simulink model "Demo_MinSegMega_V4"  (R2015a)
settings: Solver=FixedStepDiscrete  SolverMode=SingleTasking  StartTime=0.0  StopTime=inf  FixedStep=.05  RelTol=1e-3
PostLoadFcn:
  | try,
  | codertarget.arduinobase.registry.setBaudRate(gcs,115200)
  | disp('baud rate set to 115200 for external mode hardware serial')
  | baudrate='set_to_115200'
  | catch
  | disp('baud rate setting not needed in this version')
  | end
libraries: arduinolib x8, RASPlib x7, MinSegLibrary_MinSegMega x4
settings Model: SimulationMode=external  ExtModeTrigDuration=2  Creator=Alec  LastModifiedBy=hurstj
settings OptimizationCC: ExpressionDepthLimit=2147483647  OptimizeModelRefInitCode=on  LifeSpan=1
settings DebuggingCC: UnderspecifiedInitializationDetection=Classic  MergeDetectMultiDrivingBlocksExec=none  StateNameClashWarn=warning
settings HardwareCC: ProdBitPerInt=16  ProdBitPerPointer=8  ProdIntDivRoundTo=Zero  ProdEndianess=LittleEndian  ProdWordSize=8  ProdHWDeviceType=Atmel->AVR
settings RTWCC: SystemTargetFile=realtime.tlc  GenerateMakefile=off  TemplateMakefile=realtime.tmf  Description=Real-Time Toolbox  RTWVerbose=off
settings CodeAppCC: CustomSymbolStrType=$N$R$M  InternalIdentifier=Classic
settings ERTTargetCC: CombineOutputUpdateFcns=off  ExtMode=on  ExtModeTransport=3  ExtModeMexArgs=0 45 115200 30  ERTSrcFileBannerTemplate=realtime_code_template.cgt  ERTHdrFileBannerTemplate=realtime_code_template.cgt  ERTDataSrcFileTemplate=realtime_code_template.cgt  ERTDataHdrFileTemplate=realtime_code_template.cgt  ERTCustomFileTemplate=realtime_file_process.tlc

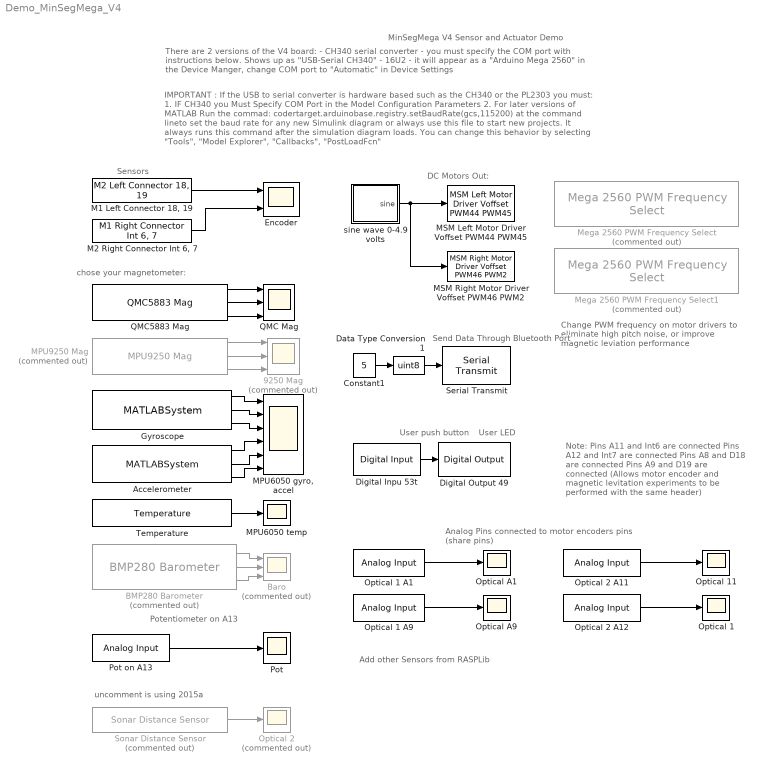
== system Demo_MinSegMega_V4 ==
  note: There are 2 versions of the V4 board:
      | - CH340 serial converter - you must specify the COM port with instructions  below. Shows up as "USB-Serial CH340"
      | - 16U2  - it will appear as a "Arduino Mega 2560" in the Device Manger, change  COM port to  "Automatic" in Device Settings
  note: Change PWM frequency on motor drivers
      | to eliminate high pitch noise, or improve
      | magnetic leviation performance
  note: Add other Sensors from RASPLib
  note: uncomment is using 2015a
  note: MinSegMega V4 Sensor and Actuator Demo
  note: DC Motors Out:
  note: Sensors
  note: Send Data Through Bluetooth Port
  note: User push button
  note: Analog Pins connected to
      | motor encoders pins (share pins)
  note: User LED
  note: Potentiometer on A13
  note: Note: Pins  A11 and Int6 are connected
      |          Pins  A12 and Int7 are connected
      | 	  Pins  A8 and D18 are connected
      |          Pins  A9 and D19 are connected
      | (Allows  motor encoder and magnetic
      | levitation experiments to be performed
      | with the same header)
  note: IMPORTANT : If the USB to serial converter is hardware based such as the CH340 or the PL2303 you must:
      | 1. IF CH340 you Must Specify COM Port in the Model Configuration Parameters
      | 2. For later versions of MATLAB Run the commad: codertarget.arduinobase.registry.setBaudRate(gcs,115200)
      | at the command lineto set the baud rate for any new Simulink diagram or always use this file to start new projects.
      | It always runs this command after the simulation diagram loads.
      | You can change this behavior by selecting "Tools", "Model Explorer", "Callbacks", "PostLoadFcn"
  note: chose your magnetometer:
  9250 Mag : Scope  Commented=on  NumInputPorts=3
      settings: TimeRange=30  YMin=-200~-200~-200  YMax=200~200~200  SaveName=ScopeData7
  Accelerometer : MATLABSystem  System=soMPU6050Accel  SimulateUsing=Code generation
      mask Type: soMPU6050Accel
      mask Display:
      | disp('soMPU6050Accel');
      | port_label('output',1,'xaccel');
      | port_label('output',2,'yaccel');
      | port_label('output',3,'zaccel');
  BMP280 Barometer : RASPlib/BMP280 Barometer  Commented=on  SimulateUsing=Code generation
  Baro : Scope  Commented=on  NumInputPorts=3
      settings: TimeRange=10  YMin=100663~53.25~28.42  YMax=100685~55.25~28.55  SaveName=ScopeData2
  Constant1 : Constant  Value=5  SampleTime=-1
  Data Type Conversion1 : DataTypeConversion  OutDataTypeStr=uint8
  Digital Inpu 53t : arduinolib/Digital Input  pinNumber=53  sampleTime=-1  blockPlatform=arduino
  Digital Output 49 : arduinolib/Digital Output  pinNumber=49  blockPlatform=arduino
  Encoder : Scope  NumInputPorts=2
      settings: TimeRange=30  YMin=-1000~-1000  YMax=1000~1000  ScrollMode=on
  Gyroscope : MATLABSystem  System=soMPU6050Gyro  DLPFmode=0
      mask Type: soMPU6050Gyro
      mask Display:
      | disp('soMPU6050Gyro');
      | port_label('output',1,'xvel');
      | port_label('output',2,'yvel');
      | port_label('output',3,'zvel');
  "M1 Left Connector 18, 19" : MinSegLibrary_MinSegMega/M2 Left Connector 18, 19  Encoder=1  PinA=19  PinB=18
  "M2 Right Connector Int 6, 7" : MinSegLibrary_MinSegMega/M1 Right Connector Int 6, 7  Encoder=2  PinA=6  PinB=7
  "MPU6050 gyro, accel" : Scope  NumInputPorts=6
      settings: TimeRange=30  YMin=-30000~-30000~-30000~-15000~-15000~-15000  YMax=30000~30000~30000~15000~15000~30000  ScrollMode=on
  MPU6050 temp : Scope
      settings: TimeRange=30  YMin=-3000  YMax=0  SaveName=ScopeData5
  MPU9250 Mag : RASPlib/MPU9250 Mag  Commented=on  SimulateUsing=Code generation
  MSM Left Motor Driver Voffset PWM44 PWM45 : MinSegLibrary_MinSegMega/MSM Left Motor Driver Voffset PWM44 PWM45  Vsupply=4.9  Voffset=0
  "MSM Right Motor Driver Voffset PWM46 PWM2 " : MinSegLibrary_MinSegMega/MSM Right Motor Driver Voffset PWM46 PWM2   Vsupply=4.9  Voffset=0
  Mega 2560 PWM Frequency Select : RASPlib/Mega 2560 PWM Frequency Select  Commented=on  Frequency=32KHz  Timer=5 - pins 44, 45, 46
  Mega 2560 PWM Frequency Select1 : RASPlib/Mega 2560 PWM Frequency Select  Commented=on  Frequency=32KHz  Timer=3 - pins 2, 3, 5
  Optical 1 : Scope
      settings: TimeRange=30  YMin=300  YMax=1100  SaveName=ScopeData8
  Optical 1 A1 : arduinolib/Analog Input  pinNumber=8  sampleTime=-1  blockPlatform=arduino
  Optical 1 A9 : arduinolib/Analog Input  pinNumber=9  sampleTime=-1  blockPlatform=arduino
  Optical 11 : Scope
      settings: TimeRange=30  YMin=300  YMax=1100  SaveName=ScopeData4
  Optical 2 : Scope  Commented=on
      settings: TimeRange=30  YMin=0  YMax=100  SaveName=ScopeData10
  Optical 2 A11 : arduinolib/Analog Input  pinNumber=11  sampleTime=-1  blockPlatform=arduino
  Optical 2 A12 : arduinolib/Analog Input  pinNumber=12  sampleTime=-1  blockPlatform=arduino
  Optical A1 : Scope
      settings: TimeRange=30  YMin=0  YMax=1000  SaveName=ScopeData9
  Optical A9 : Scope
      settings: TimeRange=30  YMin=0  YMax=1000  SaveName=ScopeData3
  Pot : Scope
      settings: TimeRange=30  YMin=0  YMax=1250  SaveName=ScopeData6  ScrollMode=on
  Pot on A13 : arduinolib/Analog Input  pinNumber=13  sampleTime=-1  blockPlatform=arduino
  QMC Mag : Scope  NumInputPorts=3
      settings: TimeRange=30  YMin=-1500~-1500~-1500  YMax=1500~1500~1500  SaveName=ScopeData11  ScrollMode=on
  QMC5883 Mag : RASPlib/QMC5883 Mag  SimulateUsing=Code generation
  Serial Transmit : arduinolib/Serial Transmit  portNumber=3  blockPlatform=arduino
  Sonar Distance Sensor : RASPlib/Sonar Distance Sensor  Commented=on  Sonar=1  TrigPin=16  EchoPin=17
  Temperature : RASPlib/Temperature  SimulateUsing=Code generation
  sine wave 0-4.9 volts : Subsystem
  wires:
  sine wave 0-4.9 volts/1(sine) -> "MSM Right Motor Driver Voffset PWM46 PWM2 "/1, MSM Left Motor Driver Voffset PWM44 PWM45/1
  Optical 1 A9/1 -> Optical A9/1
  Pot on A13/1 -> Pot/1
  Optical 2 A11/1 -> Optical 11/1
  Constant1/1 -> Data Type Conversion1/1
  Data Type Conversion1/1 -> Serial Transmit/1
  "M1 Left Connector 18, 19"/1 -> Encoder/1
  "M2 Right Connector Int 6, 7"/1 -> Encoder/2
  Optical 1 A1/1 -> Optical A1/1
  Optical 2 A12/1 -> Optical 1/1
  Sonar Distance Sensor/1 -> Optical 2/1
  Digital Inpu 53t/1 -> Digital Output 49/1
  BMP280 Barometer/1 -> Baro/1
  BMP280 Barometer/2 -> Baro/2
  Gyroscope/1 -> "MPU6050 gyro, accel"/1
  Gyroscope/2 -> "MPU6050 gyro, accel"/2
  Gyroscope/3 -> "MPU6050 gyro, accel"/3
  Accelerometer/1 -> "MPU6050 gyro, accel"/4
  Accelerometer/2 -> "MPU6050 gyro, accel"/5
  Accelerometer/3 -> "MPU6050 gyro, accel"/6
  Temperature/1 -> MPU6050 temp/1
  MPU9250 Mag/2 -> 9250 Mag/2
  MPU9250 Mag/3 -> 9250 Mag/3
  MPU9250 Mag/1 -> 9250 Mag/1
  QMC5883 Mag/2 -> QMC Mag/2
  QMC5883 Mag/3 -> QMC Mag/3
  QMC5883 Mag/1 -> QMC Mag/1
  BMP280 Barometer/3 -> Baro/3

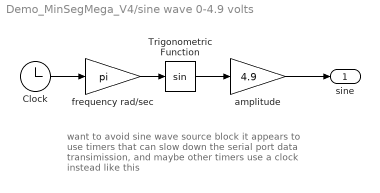
== system Demo_MinSegMega_V4/sine wave 0-4.9 volts ==
  note: want to avoid sine wave source block
      | it appears to use timers that can slow down the
      | serial port data transimission, and maybe
      | other timers
      |
      | use a clock instead like this
  Clock : Clock
  Trigonometric Function : Trigonometry
  amplitude : Gain  Gain=4.9
  frequency rad/sec : Gain  Gain=pi
  sine : Outport
  wires:
  amplitude/1 -> sine/1
  frequency rad/sec/1 -> Trigonometric Function/1
  Trigonometric Function/1 -> amplitude/1
  Clock/1 -> frequency rad/sec/1
